simulink model "Cruise"  (R2020b)
settings: Solver=ode45  StartTime=0.0  StopTime=120.0  RelTol=1e-3
undefined symbols (not defined in the file): b, M
settings Model: Creator=nadee  LastModifiedBy=nadee
settings DataIOCC: SaveOutput=off  SaveTime=off

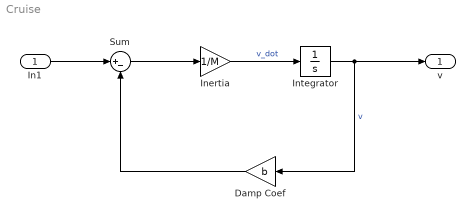
== system Cruise ==
  In1 : Inport  OutDataTypeStr=double  PortDimensions=1  SampleTime=0
  Damp Coef : Gain  Gain=b
  Inertia : Gain  Gain=1/M
  Integrator : Integrator
  Sum : Sum  Inputs=|+-
  v : Outport  OutDataTypeStr=double  PortDimensions=1  SampleTime=0
  wires:
  In1/1 -> Sum/1
  Integrator/1 -> Damp Coef/1, v/1  "v"
  Sum/1 -> Inertia/1
  Inertia/1 -> Integrator/1  "v_dot"
  Damp Coef/1 -> Sum/2
